simulink subsystem "Led_Subsystem"  (R2023b)
settings: Solver=VariableStepAuto  StartTime=0.0  StopTime=10.0  RelTol=1e-3
libraries: arduinolib x3, simulink x1
settings Model: Creator=Usuario_UMA  LastModifiedBy=javie

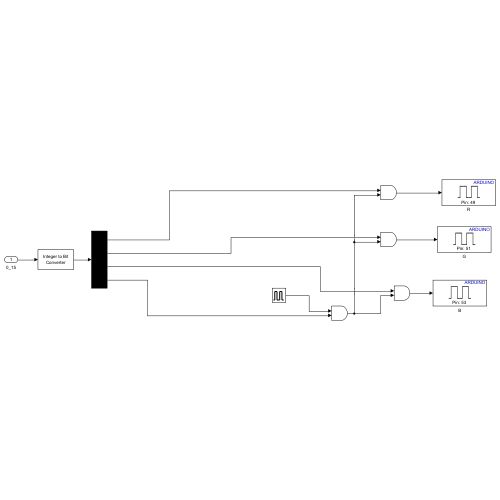
[thumbnail: Simulink's stored preview of the top-level diagram]
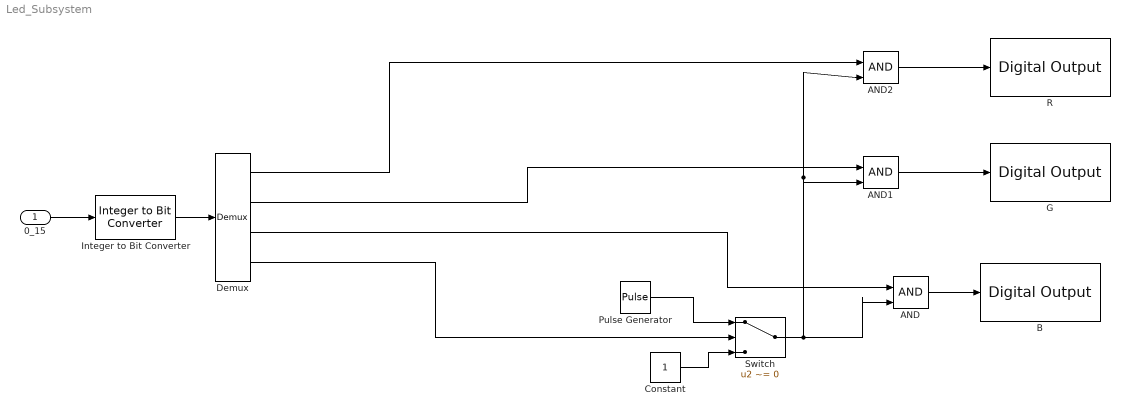
== system Led_Subsystem ==
  0_15 : Inport
  AND : Logic  IconShape=distinctive  AllPortsSameDT=off  OutDataTypeStr=boolean
  AND1 : Logic  IconShape=distinctive  AllPortsSameDT=off  OutDataTypeStr=boolean
  AND2 : Logic  IconShape=distinctive  AllPortsSameDT=off  OutDataTypeStr=boolean
  B : arduinolib/Digital Output  pinNumber=53  Direction=output  blockPlatform=arduino
  Constant : Constant
  Demux : Demux
  G : arduinolib/Digital Output  pinNumber=51  Direction=output  blockPlatform=arduino
  Integer to Bit Converter : simulink/Logic and Bit Operations/Integer to Bit Converter  nbits=4  signedInputValues=Unsigned  bitOrder=LSB first  outDtype=Inherit via internal rule
  Pulse Generator : DiscretePulseGenerator  PulseType=Time based  Period=0.5  PulseWidth=50
  R : arduinolib/Digital Output  pinNumber=49  Direction=output  blockPlatform=arduino
  Switch : Switch  Criteria=u2 ~= 0  SaturateOnIntegerOverflow=off  InputSameDT=off
  wires:
  Demux/1 -> AND2/1
  Demux/2 -> AND1/1
  Switch/1 -> AND2/2, AND1/2, AND/2
  Demux/3 -> AND/1
  AND2/1 -> R/1
  AND1/1 -> G/1
  AND/1 -> B/1
  Integer to Bit Converter/1 -> Demux/1
  0_15/1 -> Integer to Bit Converter/1
  Pulse Generator/1 -> Switch/1
  Demux/4 -> Switch/2
  Constant/1 -> Switch/3
